simulink model "current_controlled_VSC_ami8p2"  (R2017b)
settings: Solver=VariableStepDiscrete  StartTime=0.0  StopTime=0.5  FixedStep=2e-5  MaxStep=2e-5  RelTol=1e-3
InitFcn:
  | current_controlled_VSC_ami8p2_design
values from neighbouring files (symbols this model uses):
  ki = (R+Rz+ron)/taui    [current_controlled_VSC_ami8p2_design.m]
  kp = (L+Lz)/taui    [current_controlled_VSC_ami8p2_design.m]
  L = 100e-6    (= 0.0001)    [current_controlled_VSC_ami8p2_init.m]
  omega0 = 2*pi*60    (= 376.991118431)    [current_controlled_VSC_ami8p2_init.m]
  R = 0.75e-3    (= 0.00075)    [current_controlled_VSC_ami8p2_init.m]
  VDC = 1250    [current_controlled_VSC_ami8p2_init.m]
  Vn = 480    [current_controlled_VSC_ami8p2_init.m]
undefined symbols (not defined in the file or in its folder): magnitude, PLL_wmax, PLL_wmin, sigbuilder_block
libraries: powerlib x10, powerlib_meascontrol x4, cstblocks x3, simulink x2, peGeneralControl x1
settings Model: PauseTimes=0.2  Creator=divenyi  LastModifiedBy=divenyi

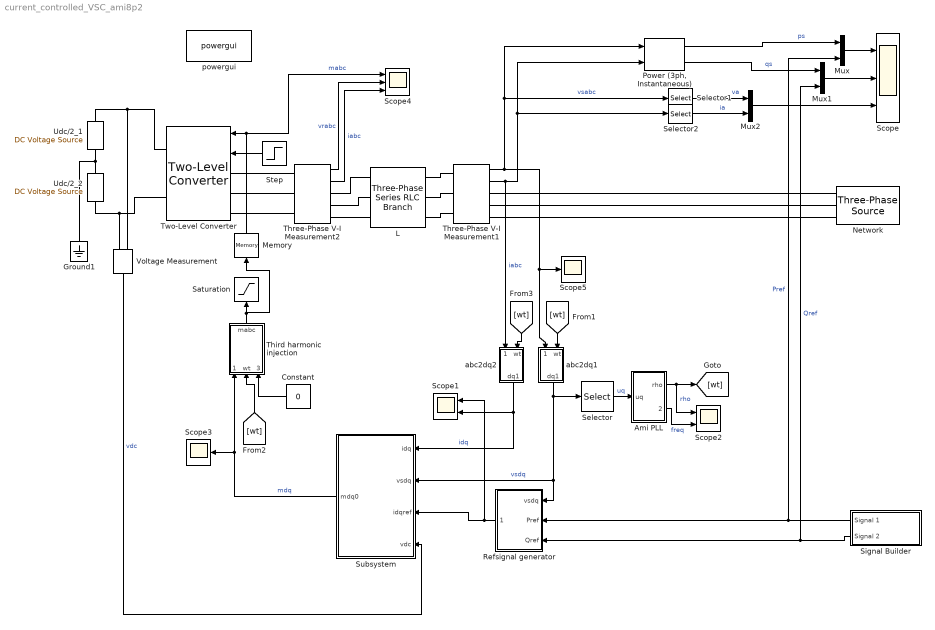
== system current_controlled_VSC_ami8p2 ==
  Ami PLL : Subsystem
  Constant : Constant  Value=0
  Ground1 : powerlib/Elements/Ground  LConnTagsString=a
  L : powerlib/Elements/Three-Phase Series RLC Branch  LConnTagsString=A|B|C  RConnTagsString=A|B|C  BranchType=RL  Resistance=R  Inductance=L  Capacitance=1e-6  Measurements=None
  Memory : Memory
  Mux : Mux  Inputs=2
  Mux1 : Mux  Inputs=2
  Mux2 : Mux  Inputs=2
  Network : powerlib/Electrical Sources/Three-Phase Source  InternalConnection=Yg  VoltagePhases=off  Voltage=Vn  PhaseAngle=0  Voltage_phases=[25e3 25e3 25e3]/sqrt(3)  PhaseAngles_phases=[0 -120 +120]  Frequency=omega0/2/pi  NonIdealSource=off  SpecifyImpedance=on  Resistance=10  Inductance=0  ShortCircuitLevel=Sz  BaseVoltage=Un  XRratio=X_R_ratio  BusType=swing  Pref=10e3  Qref=0  Prefabc=[10e3, 10e3, 10e3]  Qrefabc=[0, 0, 0]  Qmin=-inf  Qmax=inf
  "Power (3ph, Instantaneous)" : powerlib_meascontrol/Measurements/Power (3ph, Instantaneous)
      settings: SourceProductName=Simscape Power Systems
  Refsignal generator : Subsystem
  Saturation : Saturate  UpperLimit=1  LowerLimit=-1
  Scope : Scope  NumInputPorts=3
  Scope1 : Scope  NumInputPorts=2
  Scope2 : Scope  NumInputPorts=2
  Scope3 : Scope
  Scope4 : Scope  NumInputPorts=3
  Scope5 : Scope
  Selector : Selector  InputPortWidth=2  IndexOptions=Index vector (dialog)  Indices=[2]  OutputSizes=1
  Selector1 : Selector  InputPortWidth=3  IndexOptions=Index vector (dialog)  Indices=[1]  OutputSizes=1
  Selector2 : Selector  InputPortWidth=3  IndexOptions=Index vector (dialog)  Indices=[1]  OutputSizes=1
  Signal Builder : Subsystem  Tag=STV Subsys  LoadFcn=sigbuilder_block('load');  StartFcn=sigbuilder_block('start');  StopFcn=sigbuilder_block('stop');  ClipboardFcn=sigbuilder_block('clipboard');  mask(Sigbuilder block){tuvar=[0:10]}
      mask help: Simulink:masks:SigbuilderBlock_MD
      mask init:
      | if ~strcmp(get_param(bdroot(gcbh),'SimulationStatus'),'stopped') tuvar = sigbuilder_block('maskInit'); end
      settings: CopyFcn=sigbuilder_block('copy');  DeleteFcn=sigbuilder_block('delete');  ModelCloseFcn=sigbuilder_block('modelClose');  PreSaveFcn=sigbuilder_block('preSave');  PauseFcn=sigbuilder_block('pause');  ContinueFcn=sigbuilder_block('continue');  NameChangeFcn=sigbuilder_block('namechange');  OpenFcn=sigbuilder_block('open',[437.6 199.2 550.4 400 ]);  CloseFcn=sigbuilder_block('close');
      mask Display: plot(0, 0, 100, 100,[2, 2, 32, 32, 2], [68, 8, 8, 68, 68],[32, 2], [38, 38], [32, 19, 2],[53, 60, 44], [32, 17, 17, 2],[16, 16, 31, 31]);txt = getActiveGroup(gcbh);text(2, 100, txt,'verticalAlignment', 'top');
  Step : Step  Time=0.15  Before=1  After=0  SampleTime=0
  Subsystem : Subsystem
  "Third harmonic injection " : Subsystem
  Three-Phase V-I Measurement1 : powerlib/Measurements/Three-Phase V-I Measurement  VoltageMeasurement=phase-to-ground  SetLabelV=off  LabelV=Vabc  Vpu=off  VpuLL=off  CurrentMeasurement=yes  SetLabelI=off  LabelI=Iabc  Ipu=off  Pbase=100e6  Vbase=500e3  OutputType=Complex  PhasorSimulation=off  PSBequivalent=0
  Three-Phase V-I Measurement2 : powerlib/Measurements/Three-Phase V-I Measurement  VoltageMeasurement=phase-to-ground  SetLabelV=off  LabelV=Vabc  Vpu=off  VpuLL=off  CurrentMeasurement=yes  SetLabelI=off  LabelI=Iabc  Ipu=off  Pbase=100e6  Vbase=500e3  OutputType=Complex  PhasorSimulation=off  PSBequivalent=0
  Two-Level Converter : powerlib/Power Electronics/Two-Level Converter  ModelType=Average model (Uref-controlled)  Ron=ron  Rs=1e6  Cs=inf  Vforward=[0,0]  Ron_Diode=ron  Rs_Diode=1e6  Cs_Diode=inf  Vf_Diode=Vd  Rs_CurrentSource=inf
      settings: SourceProductName=Simscape Power Systems  SourceProductBaseCode=PS
  Udc/2_1 : powerlib/Electrical Sources/DC Voltage Source  Amplitude=VDC/2  Measurements=None
  Udc/2_2 : powerlib/Electrical Sources/DC Voltage Source  Amplitude=VDC/2  Measurements=None
  Voltage Measurement : powerlib/Measurements/Voltage Measurement  PhasorSimulation=off  OutputType=Complex  PSBequivalent=0
  abc2dq1 : Subsystem
  abc2dq2 : Subsystem
  powergui : powerlib/powergui  Priority=1  SimulationMode=Discrete  SampleTime=1e-6  frequency=60  Iterations=50  frequencyindice=0  Pbase=100e6  ErrMax=1e-4  UnitsV=kV  UnitsW=MW  buscounter=0  FunctionMessages=off  echomessages=off  EnableUseOfTLC=off  CurrentSourceSwitches=off  DisableSnubberDevices=off  DisableRonSwitches=off  DisableVfSwitches=off  DisplayEquations=off  SolverType=Tustin/Backward Euler (TBE)  Interpol=off  ExternalGateDelay=off  methode=off  Ts=100  x0status=blocks  SPID=on  SwTol=0  HookPort=off  RestoreLinks=warning  ResistiveCurrentMeasurement=off  Frange=[0:2:500]  Ylog=off  Xlog=on  ShowGrid=off  save=off  variable=ZData  structure=0  ZoomFFT=off  StartTime=0.0  cycles=1  DisplayStyle=1  fundamental=60  FreqAxis=off  MaxFrequency=1000  frequencyindicesteady=1  RmsSteady=1  display=off
  wires:
  Three-Phase V-I Measurement1/1 -> Scope5/1, abc2dq1/1(abc), "Power (3ph, Instantaneous)"/1, Selector1/1  "vsabc"
  Ami PLL/1(rho) -> Scope2/1, [wt]  "rho"
  Signal Builder/1(Signal 1) -> Refsignal generator/2(Pref), Mux/2  "Pref"
  Signal Builder/2(Signal 2) -> Mux1/2, Refsignal generator/3(Qref)  "Qref"
  Refsignal generator/1(idqref) -> Scope1/1, Subsystem/3(idqref)
  Voltage Measurement/1 -> Subsystem/4(vdc)  "vdc"
  Three-Phase V-I Measurement1/2 -> abc2dq2/1(abc), "Power (3ph, Instantaneous)"/2, Selector2/1  "iabc"
  abc2dq1/1(dq1) -> Selector/1, Subsystem/2(vsdq), Refsignal generator/1(vsdq)  "vsdq"
  Selector/1 -> Ami PLL/1(uq)  "uq"
  abc2dq2/1(dq1) -> Scope1/2, Subsystem/1(idq)  "idq"
  "Power (3ph, Instantaneous)"/1 -> Mux/1  "ps"
  Mux/1 -> Scope/1
  Mux1/1 -> Scope/2
  "Power (3ph, Instantaneous)"/2 -> Mux1/1  "qs"
  Mux2/1 -> Scope/3
  Selector1/1 -> Mux2/1  "va"
  Selector2/1 -> Mux2/2  "ia"
  [wt] -> abc2dq1/2(wt)
  [wt] -> abc2dq2/2(wt)
  Step/1 -> Two-Level Converter/2
  Ami PLL/2(freq) -> Scope2/2  "freq"
  Three-Phase V-I Measurement2/1 -> Scope4/2  "vrabc"
  Three-Phase V-I Measurement2/2 -> Scope4/3  "iabc"
  Subsystem/1(mdq0) -> "Third harmonic injection "/1(mdq), Scope3/1  "mdq"
  Memory/1 -> Scope4/1, Two-Level Converter/1  "mabc"
  "Third harmonic injection "/1(mabc) -> Memory/1, Saturation/1
  [wt] -> "Third harmonic injection "/2(wt)
  Constant/1 -> "Third harmonic injection "/3(enable)
  connections:
  L/RConn1 -- Three-Phase V-I Measurement1/LConn1
  L/RConn2 -- Three-Phase V-I Measurement1/LConn2
  Three-Phase V-I Measurement1/LConn3 -- L/RConn3
  Udc/2_2/RConn1 -- Ground1/LConn1 -- Udc/2_1/LConn1
  Udc/2_2/LConn1 -- Two-Level Converter/RConn2 -- Voltage Measurement/LConn2
  Three-Phase V-I Measurement1/RConn3 -- Network/RConn3
  Three-Phase V-I Measurement1/RConn2 -- Network/RConn2
  Three-Phase V-I Measurement1/RConn1 -- Network/RConn1
  Udc/2_1/RConn1 -- Two-Level Converter/RConn1 -- Voltage Measurement/LConn1
  Three-Phase V-I Measurement2/RConn1 -- L/LConn1
  Three-Phase V-I Measurement2/RConn2 -- L/LConn2
  Three-Phase V-I Measurement2/RConn3 -- L/LConn3
  Three-Phase V-I Measurement2/LConn2 -- Two-Level Converter/LConn2
  Three-Phase V-I Measurement2/LConn3 -- Two-Level Converter/LConn3
  Three-Phase V-I Measurement2/LConn1 -- Two-Level Converter/LConn1

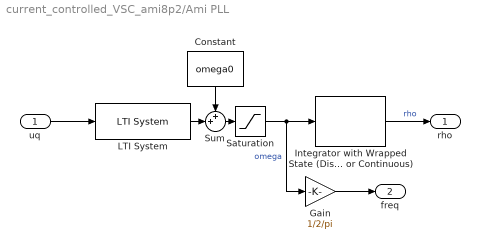
== system current_controlled_VSC_ami8p2/Ami PLL ==
  uq : Inport
  Constant : Constant  Value=omega0
  Gain : Gain  Gain=1/2/pi
  Integrator with Wrapped State (Discrete or Continuous) : peGeneralControl/Integrator with Wrapped State (Discrete or Continuous)  OverrideUsingVariant=Discrete  WrappedStateUpperValue=2*pi  WrappedStateLowerValue=0  x0=0  Ts=-1
  LTI System : cstblocks/LTI System  sys=PLL_H  IC=[]
  Saturation : Saturate  UpperLimit=PLL_wmax  LowerLimit=PLL_wmin
  Sum : Sum  Inputs=++|
  rho : Outport
  freq : Outport  Port=2
  wires:
  Saturation/1 -> Gain/1, Integrator with Wrapped State (Discrete or Continuous)/1  "omega"
  Integrator with Wrapped State (Discrete or Continuous)/1 -> rho/1  "rho"
  uq/1 -> LTI System/1
  Gain/1 -> freq/1
  LTI System/1 -> Sum/2
  Sum/1 -> Saturation/1
  Constant/1 -> Sum/1

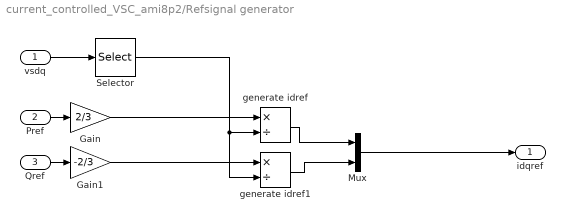
== system current_controlled_VSC_ami8p2/Refsignal generator ==
  vsdq : Inport
  Pref : Inport  Port=2
  Qref : Inport  Port=3
  Gain : Gain  Gain=2/3
  Gain1 : Gain  Gain=-2/3
  Mux : Mux  Inputs=2
  Selector : Selector  InputPortWidth=2  IndexOptions=Index vector (dialog)  Indices=[1]  OutputSizes=1
  generate idref : Product  Inputs=*/
  generate idref1 : Product  Inputs=*/
  idqref : Outport
  wires:
  Gain/1 -> generate idref/1
  Pref/1 -> Gain/1
  Qref/1 -> Gain1/1
  Gain1/1 -> generate idref1/1
  vsdq/1 -> Selector/1
  generate idref/1 -> Mux/1
  generate idref1/1 -> Mux/2
  Selector/1 -> generate idref/2, generate idref1/2
  Mux/1 -> idqref/1

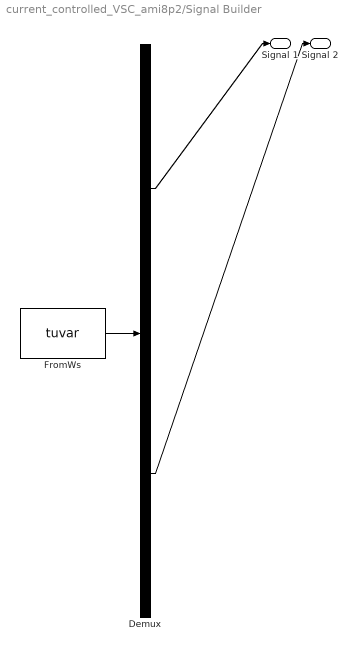
== system current_controlled_VSC_ami8p2/Signal Builder ==
  Demux : Demux  Tag=STV Demux  Outputs=2
  FromWs : FromWorkspace  Tag=STV FromWs  VariableName=tuvar  SampleTime=0
      SigBuilderData=|
      | common.afterFinalStr = 'Extrapolate'
      | common.sampleTime = 0
      | dataSet.timeRange = [0 0.5]
      | dataSet.name = 'Group 1'
      | sbobj.Groups.Name = 'Group 1'
      | sbobj.Groups.Signals(1).Name = 'Signal 1'
      | sbobj.Groups.Signals(1).XData = [0 0.2 0.2 0.3 0.3 0.5]
      | sbobj.Groups.Signals(1).YData = [0 0 2500000 2500000 -2500000 -2500000]
      | sbobj.Groups.Signals(2).Name = 'Signal 2'
      | sbobj.Groups.Signals(2).XData = [0 0.35 0.35 0.5]
      | sbobj.Groups.Signals(2).YData = [100 100 1000000 1000000]
      | sbobj.Groups.TimeRange = [0 0.5]
  Signal 1 : Outport  Tag=STV Outport
  Signal 2 : Outport  Tag=STV Outport  Port=2
  wires:
  Demux/1 -> Signal 1/1
  FromWs/1 -> Demux/1
  Demux/2 -> Signal 2/1

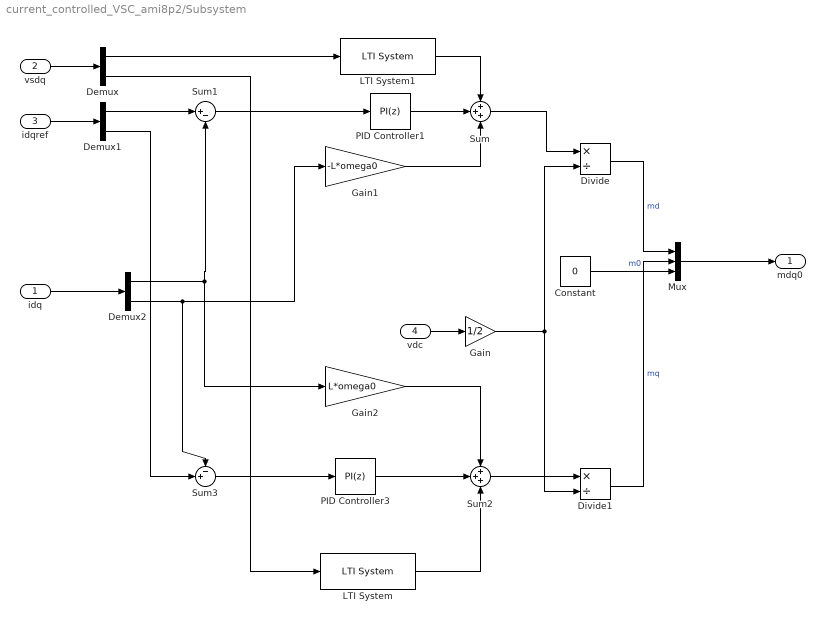
== system current_controlled_VSC_ami8p2/Subsystem ==
  idq : Inport
  vsdq : Inport  Port=2
  idqref : Inport  Port=3
  vdc : Inport  Port=4
  Constant : Constant  Value=0
  Demux : Demux  Outputs=2
  Demux1 : Demux  Outputs=2
  Demux2 : Demux  Outputs=2
  Divide : Product  Inputs=*/
  Divide1 : Product  Inputs=*/
  Gain : Gain  Gain=1/2
  Gain1 : Gain  Gain=-L*omega0
  Gain2 : Gain  Gain=L*omega0
  LTI System : cstblocks/LTI System  sys=Gff  IC=[]
  LTI System1 : cstblocks/LTI System  sys=Gff  IC=[]
  Mux : Mux  Inputs=3
  PID Controller1 : simulink/Continuous/PID Controller  Controller=PI  TimeDomain=Discrete-time  SampleTime=-1  IntegratorMethod=Forward Euler  FilterMethod=Forward Euler  Form=Parallel  UseFilter=on  ControllerParametersSource=internal  P=kp  I=ki  D=0  N=100  InitialConditionSource=internal  InitialConditionForIntegrator=0  InitialConditionForFilter=0  ExternalReset=none  LimitOutput=off  UpperSaturationLimit=inf  LowerSaturationLimit=-inf  LinearizeAsGain=on  AntiWindupMode=none  Kb=1  TrackingMode=off  Kt=1  PParamMin=[]  PParamMax=[]  IParamMin=[]  IParamMax=[]  DParamMin=[]  DParamMax=[]  NParamMin=[]  NParamMax=[]  KbParamMin=[]  KbParamMax=[]  KtParamMin=[]  KtParamMax=[]  POutMin=[]  POutMax=[]  IOutMin=[]  IOutMax=[]  DOutMin=[]  DOutMax=[]  NOutMin=[]  NOutMax=[]  KbOutMin=[]  KbOutMax=[]  KtOutMin=[]  KtOutMax=[]  IntegratorOutMin=[]  IntegratorOutMax=[]  FilterOutMin=[]  FilterOutMax=[]  SumOutMin=[]  SumOutMax=[]  SumI1OutMin=[]  SumI1OutMax=[]  SumI2OutMin=[]  SumI2OutMax=[]  SumI3OutMin=[]  SumI3OutMax=[]  SumDOutMin=[]  SumDOutMax=[]  SaturationOutMin=[]  SaturationOutMax=[]  IntegratorContinuousStateAttributes=''  IntegratorStateMustResolveToSignalObject=off  IntegratorRTWStateStorageClass=Auto  FilterContinuousStateAttributes=''  FilterStateMustResolveToSignalObject=off  FilterRTWStateStorageClass=Auto  DifferentiatorICPrevScaledInput=0  DifferentiatorOutMin=[]  DifferentiatorOutMax=[]  InitialConditionSetting=State (most efficient)  FilterDiffOutCoefMin=[]  FilterDiffOutCoefMax=[]  SumDenOutMin=[]  SumDenOutMax=[]  SumNumOutMin=[]  SumNumOutMax=[]  ReciprocalOutMin=[]  ReciprocalOutMax=[]  DivideOutMin=[]  DivideOutMax=[]  TunerSelectOption=Transfer Function Based (PID Tuner App)
  PID Controller3 : simulink/Continuous/PID Controller  Controller=PI  TimeDomain=Discrete-time  SampleTime=-1  IntegratorMethod=Forward Euler  FilterMethod=Forward Euler  Form=Parallel  UseFilter=on  ControllerParametersSource=internal  P=kp  I=ki  D=0  N=100  InitialConditionSource=internal  InitialConditionForIntegrator=0  InitialConditionForFilter=0  ExternalReset=none  LimitOutput=off  UpperSaturationLimit=inf  LowerSaturationLimit=-inf  LinearizeAsGain=on  AntiWindupMode=none  Kb=1  TrackingMode=off  Kt=1  PParamMin=[]  PParamMax=[]  IParamMin=[]  IParamMax=[]  DParamMin=[]  DParamMax=[]  NParamMin=[]  NParamMax=[]  KbParamMin=[]  KbParamMax=[]  KtParamMin=[]  KtParamMax=[]  POutMin=[]  POutMax=[]  IOutMin=[]  IOutMax=[]  DOutMin=[]  DOutMax=[]  NOutMin=[]  NOutMax=[]  KbOutMin=[]  KbOutMax=[]  KtOutMin=[]  KtOutMax=[]  IntegratorOutMin=[]  IntegratorOutMax=[]  FilterOutMin=[]  FilterOutMax=[]  SumOutMin=[]  SumOutMax=[]  SumI1OutMin=[]  SumI1OutMax=[]  SumI2OutMin=[]  SumI2OutMax=[]  SumI3OutMin=[]  SumI3OutMax=[]  SumDOutMin=[]  SumDOutMax=[]  SaturationOutMin=[]  SaturationOutMax=[]  IntegratorContinuousStateAttributes=''  IntegratorStateMustResolveToSignalObject=off  IntegratorRTWStateStorageClass=Auto  FilterContinuousStateAttributes=''  FilterStateMustResolveToSignalObject=off  FilterRTWStateStorageClass=Auto  DifferentiatorICPrevScaledInput=0  DifferentiatorOutMin=[]  DifferentiatorOutMax=[]  InitialConditionSetting=State (most efficient)  FilterDiffOutCoefMin=[]  FilterDiffOutCoefMax=[]  SumDenOutMin=[]  SumDenOutMax=[]  SumNumOutMin=[]  SumNumOutMax=[]  ReciprocalOutMin=[]  ReciprocalOutMax=[]  DivideOutMin=[]  DivideOutMax=[]  TunerSelectOption=Transfer Function Based (PID Tuner App)
  Sum : Sum  Inputs=+++
  Sum1 : Sum  Inputs=|+-
  Sum2 : Sum  Inputs=+++
  Sum3 : Sum  Inputs=-+|
  mdq0 : Outport
  wires:
  vdc/1 -> Gain/1
  Gain/1 -> Divide1/2, Divide/2
  Sum/1 -> Divide/1
  Divide/1 -> Mux/1  "md"
  Constant/1 -> Mux/3  "m0"
  Mux/1 -> mdq0/1
  vsdq/1 -> Demux/1
  idqref/1 -> Demux1/1
  Demux1/1 -> Sum1/1
  idq/1 -> Demux2/1
  Gain1/1 -> Sum/3
  Gain2/1 -> Sum2/1
  Demux2/1 -> Gain2/1, Sum1/2
  Demux2/2 -> Gain1/1, Sum3/1
  Demux1/2 -> Sum3/2
  PID Controller3/1 -> Sum2/2
  Sum3/1 -> PID Controller3/1
  Sum2/1 -> Divide1/1
  Divide1/1 -> Mux/2  "mq"
  Demux/2 -> LTI System/1
  Demux/1 -> LTI System1/1
  Sum1/1 -> PID Controller1/1
  PID Controller1/1 -> Sum/2
  LTI System/1 -> Sum2/3
  LTI System1/1 -> Sum/1

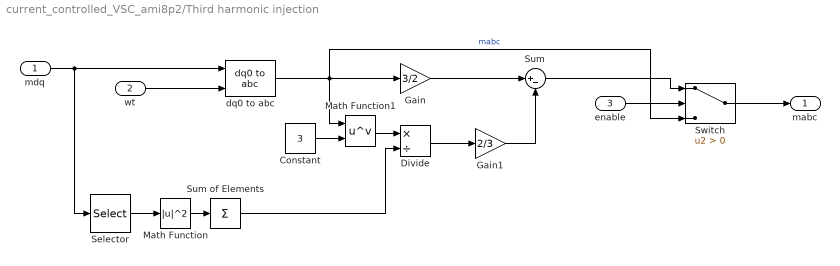
== system current_controlled_VSC_ami8p2/Third harmonic injection  ==
  mdq : Inport
  wt : Inport  Port=2
  enable : Inport  Port=3
  Constant : Constant  Value=3
  Divide : Product  Inputs=*/
  Gain : Gain  Gain=3/2
  Gain1 : Gain  Gain=2/3
  Math Function : Math  Operator=magnitude^2  SaturateOnIntegerOverflow=on
  Math Function1 : Math  Operator=pow  SaturateOnIntegerOverflow=on
  Selector : Selector  InputPortWidth=3  IndexOptions=Index vector (dialog)  Indices=[1 2]  OutputSizes=1
  Sum : Sum  Inputs=|+-
  Sum of Elements : Sum  Inputs=+
  Switch : Switch  Criteria=u2 > Threshold
  dq0 to abc : powerlib_meascontrol/Transformations/dq0 to abc  Alignment=90 degrees behind phase A axis
  mabc : Outport
  wires:
  dq0 to abc/1 -> Switch/3, Math Function1/1, Gain/1  "mabc"
  wt/1 -> dq0 to abc/2
  mdq/1 -> Selector/1, dq0 to abc/1
  Selector/1 -> Math Function/1
  Math Function/1 -> Sum of Elements/1
  Constant/1 -> Math Function1/2
  Math Function1/1 -> Divide/1
  Sum of Elements/1 -> Divide/2
  Divide/1 -> Gain1/1
  Gain/1 -> Sum/1
  Gain1/1 -> Sum/2
  Switch/1 -> mabc/1
  enable/1 -> Switch/2
  Sum/1 -> Switch/1

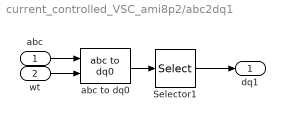
== system current_controlled_VSC_ami8p2/abc2dq1 ==
  abc : Inport
  wt : Inport  Port=2
  Selector1 : Selector  InputPortWidth=3  IndexOptions=Index vector (dialog)  Indices=[1 2]  OutputSizes=1
  abc to dq0 : powerlib_meascontrol/Transformations/abc to dq0  Alignment=90 degrees behind phase A axis
  dq1 : Outport
  wires:
  abc to dq0/1 -> Selector1/1
  Selector1/1 -> dq1/1
  abc/1 -> abc to dq0/1
  wt/1 -> abc to dq0/2

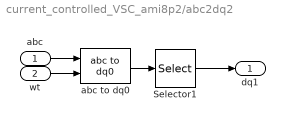
== system current_controlled_VSC_ami8p2/abc2dq2 ==
  abc : Inport
  wt : Inport  Port=2
  Selector1 : Selector  InputPortWidth=3  IndexOptions=Index vector (dialog)  Indices=[1 2]  OutputSizes=1
  abc to dq0 : powerlib_meascontrol/Transformations/abc to dq0  Alignment=90 degrees behind phase A axis
  dq1 : Outport
  wires:
  wt/1 -> abc to dq0/2
  abc/1 -> abc to dq0/1
  Selector1/1 -> dq1/1
  abc to dq0/1 -> Selector1/1
